simulink model "Aenea_model"  (R2020b)
settings: Solver=FixedStepDiscrete  StartTime=0.0  StopTime=10.0  FixedStep=0.02  RelTol=1e-3
undefined symbols (not defined in the file or in its folder): attuatore_Amax, attuatore_Amin, attuatore_Emax, attuatore_Emin, attuatore_Rmax, attuatore_Rmin, attuatore_Tmax, attuatore_Tmin, bias, DiscIntNeverNeededParam, interventoA_05, interventoA_1, interventoE_05, interventoE_1, interventoT, inv_A, inv_comp_h, inv_E, inv_R, inv_T, K_AW_B_AP_quota, K_AW_B_becc, K_AW_B_imb, K_AW_B_roll, K_imb_inv, Kd_h_app, Kd_h_flare, Ki_AP_quota_select, Ki_AP_rotta, Ki_AP_vel, Ki_becch, Ki_h_app, Ki_h_cruise, Ki_h_flare, Ki_roll, Kp_AP_quota_hold_h, Kp_AP_quota_hold_l, Kp_AP_quota_select, Kp_AP_rotta, Kp_AP_vel, Kp_becch, Kp_comp_h, Kp_h_app_max, Kp_h_app_min, Kp_h_cruise, Kp_h_flare, Kp_imb, Kp_p, Kp_q, Kp_roll, Kp_Rotta_ATO, Newton, phi_max, phi_min, Q1B, R1B, Raphson, safe_phi, safe_V, Sensor_Offsets ... (+11)
libraries: simulink_extras x41, slpidlib x8, simulink x6, dspsigops x4, arduinolib x3, svdutilitieslib x3, aerolibtransform2sys x2, aerolibtransform2 x2, aerosimlib x2, cstblocks x1
(part 4 of 7)

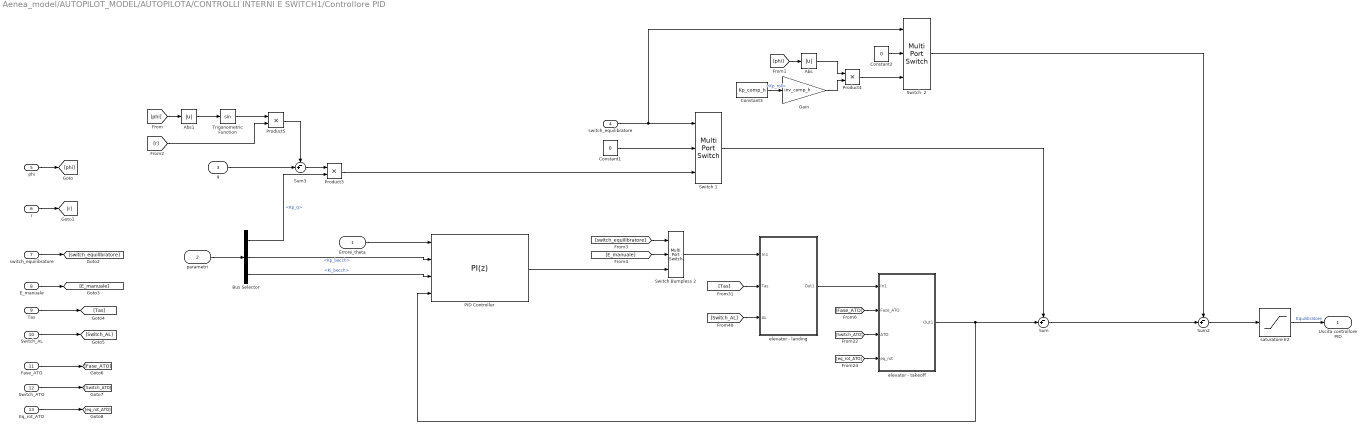
== system Aenea_model/AUTOPILOT_MODEL/AUTOPILOTA/CONTROLLI INTERNI E SWITCH1/Controllore PID ==
  Errore_theta : Inport
  parametri : Inport  Port=2
  "q " : Inport  Port=3
  "switch_equilibratore " : Inport  Port=4
  "phi " : Inport  Port=5
  r : Inport  Port=6
  switch_equilibratore : Inport  Port=7
  E_manuale : Inport  Port=8
  Tas : Inport  Port=9
  Switch_AL : Inport  Port=10
  Fase_ATO : Inport  Port=11
  Switch_ATO : Inport  Port=12
  Eq_rot_ATO : Inport  Port=13
  Abs : Abs
  Abs1 : Abs
  Bus Selector : BusSelector  OutputSignals=Kp_q,Kp_becch,Ki_becch
  Constant1 : Constant  Value=0  SampleTime=0.02
  Constant2 : Constant  Value=0  SampleTime=0.02
  Constant3 : Constant  Value=Kp_comp_h  SampleTime=0.02
  Gain : Gain  Gain=inv_comp_h
  PID Controller : slpidlib/PID Controller  Controller=PI  Form=Parallel  TimeDomain=Discrete-time  UseExternalTs=off  SampleTime=-1  IntegratorMethod=Forward Euler  FilterMethod=Forward Euler  ControllerParametersSource=external  P=1  I=1  D=1  UseFilter=off  N=100  TunerSelectOption=Transfer Function Based (PID Tuner App)  InitialConditionSource=internal  InitialConditionForIntegrator=0  InitialConditionForFilter=0  DifferentiatorICPrevScaledInput=0  ExternalReset=none  TrackingMode=on  Kt=1  LimitOutput=on  SatLimitsSource=internal  UpperSaturationLimit=attuatore_Emax  LowerSaturationLimit=attuatore_Emin  LinearizeAsGain=on  AntiWindupMode=back-calculation  Kb=1  POutMin=[]  POutMax=[]  IOutMin=[]  IOutMax=[]  DOutMin=[]  DOutMax=[]  NOutMin=[]  NOutMax=[]  SumOutMin=[]  SumOutMax=[]  SaturationOutMin=[]  SaturationOutMax=[]  PParamMin=[]  PParamMax=[]  IParamMin=[]  IParamMax=[]  DParamMin=[]  DParamMax=[]  NParamMin=[]  NParamMax=[]  KbParamMin=[]  KbParamMax=[]  KtParamMin=[]  KtParamMax=[]  KbOutMin=[]  KbOutMax=[]  KtOutMin=[]  KtOutMax=[]  IntegratorOutMin=[]  IntegratorOutMax=[]  FilterOutMin=[]  FilterOutMax=[]  SumI1OutMin=[]  SumI1OutMax=[]  SumI2OutMin=[]  SumI2OutMax=[]  SumI3OutMin=[]  SumI3OutMax=[]  SumI4OutMin=[]  SumI4OutMax=[]  SumDOutMin=[]  SumDOutMax=[]  DifferentiatorOutMin=[]  DifferentiatorOutMax=[]  FilterDiffOutCoefMin=[]  FilterDiffOutCoefMax=[]  ReciprocalOutMin=[]  ReciprocalOutMax=[]  SumDenOutMin=[]  SumDenOutMax=[]  SumNumOutMin=[]  SumNumOutMax=[]  DivideOutMin=[]  DivideOutMax=[]  UdiffTsProdOutMin=[]  UdiffTsProdOutMax=[]  NTsProdOutMin=[]  NTsProdOutMax=[]  UintegralTsProdOutMin=[]  UintegralTsProdOutMax=[]  UngainTsProdOutMin=[]  UngainTsProdOutMax=[]  IntegratorContinuousStateAttributes=''  IntegratorStateMustResolveToSignalObject=off  IntegratorRTWStateStorageClass=Auto  FilterContinuousStateAttributes=''  FilterStateMustResolveToSignalObject=off  FilterRTWStateStorageClass=Auto  ParallelPVariant=ExternalParameters  IdealPVariant=Disabled  IVariant=ExternalParameters  DVariant=Disabled  IntegratorVariant=Discrete  SatVariant=Enabled  AWVariant=BackCalculation  PCopyVariant=Disabled  TRVariant=Enabled  FdbkBlocksVariant=Forward  IdealPFdbkVariant=Disabled  SatFdbkVariant=Disabled  DerivativeFilterVariant=Disabled  NVariant=Disabled  NCopyVariant=Disabled_SignalSpec  FilterICVariant=Disabled  IntegratorICVariant=InternalICs  ExternalResetVariant=Disabled  TRSumVariant=TrackingMode  SumFdbkVariant=Disabled  SumVariant=Sum_PI  TsampFilterVariant=InternalTs  TsampNgainVariant=Passthrough  TsampIntegralVariant=Passthrough  ExternalSaturationOutDataTypeStr=Inherit: Same as second input
  Product3 : Product  RndMeth=Zero
  Product4 : Product  RndMeth=Zero
  Product5 : Product  RndMeth=Zero
  Sum : Sum  Inputs=-+|
  Sum2 : Sum  Inputs=-+|
  Sum3 : Sum  Inputs=-+|
  Switch  2 : MultiPortSwitch  DataPortOrder=Zero-based contiguous  Inputs=2  zeroidx=on
  Switch 1 : MultiPortSwitch  DataPortOrder=Zero-based contiguous  Inputs=2  zeroidx=on
  Switch Bumpless 2 : MultiPortSwitch  DataPortOrder=Zero-based contiguous  Inputs=2  zeroidx=on
  Trigonometric Function : Trigonometry
  elevator - landing : Subsystem
  elevator - takeoff : Subsystem
  saturatore E2 : Saturate  UpperLimit=attuatore_Emax  LowerLimit=attuatore_Emin
  Uscita controllore PID : Outport  VectorParamsAs1DForOutWhenUnconnected=off
  wires:
  Errore_theta/1 -> PID Controller/1
  parametri/1 -> Bus Selector/1
  Bus Selector/2 -> PID Controller/2  "<Kp_becch>"
  Bus Selector/3 -> PID Controller/3  "<Ki_becch>"
  Bus Selector/1 -> Product3/2  "<Kp_q>"
  Switch 1/1 -> Sum/1
  Product3/1 -> Switch 1/3
  Constant1/1 -> Switch 1/2
  elevator - takeoff/1(Out1) -> PID Controller/4, Sum/2
  Sum2/1 -> saturatore E2/1
  [phi] -> Abs/1
  Switch  2/1 -> Sum2/1
  Product4/1 -> Switch  2/3
  Constant2/1 -> Switch  2/2
  "switch_equilibratore "/1 -> Switch  2/1, Switch 1/1
  Abs/1 -> Product4/1
  [phi] -> Abs1/1
  Abs1/1 -> Trigonometric Function/1
  "phi "/1 -> [phi]
  r/1 -> [r]
  Trigonometric Function/1 -> Product5/1
  [r] -> Product5/2
  "q "/1 -> Sum3/2
  Sum3/1 -> Product3/1
  Product5/1 -> Sum3/1
  Sum/1 -> Sum2/2
  Switch Bumpless 2/1 -> elevator - landing/1(In1)
  Gain/1 -> Product4/2
  [Tas] -> elevator - landing/2(Tas)
  [Switch_AL] -> elevator - landing/3(AL)
  [Switch_ATO] -> elevator - takeoff/3(ATO)
  [Fase_ATO] -> elevator - takeoff/2(Fase_ATO)
  [eq_rot_ATO] -> elevator - takeoff/4(eq_rot)
  elevator - landing/1(Out1) -> elevator - takeoff/1(In1)
  [E_manuale] -> Switch Bumpless 2/2
  PID Controller/1 -> Switch Bumpless 2/3
  [switch_equilibratore] -> Switch Bumpless 2/1
  switch_equilibratore/1 -> [switch_equilibratore]
  E_manuale/1 -> [E_manuale]
  Tas/1 -> [Tas]
  Switch_AL/1 -> [Switch_AL]
  Fase_ATO/1 -> [Fase_ATO]
  Switch_ATO/1 -> [Switch_ATO]
  Eq_rot_ATO/1 -> [eq_rot_ATO]
  saturatore E2/1 -> Uscita controllore PID/1  "Equilibratore"
  Constant3/1 -> Gain/1  "<Kp_roll>"

== system Aenea_model/AUTOPILOT_MODEL/AUTOPILOTA/CONTROLLI INTERNI E SWITCH1/Controllore PID1 ==
  Err_Trk : Inport
  Errore_phi : Inport  Port=2
  parametri : Inport  Port=3
  "p " : Inport  Port=4
  "switch_alettoni " : Inport  Port=5
  Fase_ATO : Inport  Port=6
  Bus Selector : BusSelector  OutputSignals=Kp_p,Kp_roll,Ki_roll
  Constant1 : Constant  Value=0  SampleTime=0.02
  Constant3 : Constant  Value=2
  PID Controller : slpidlib/PID Controller  Controller=PI  Form=Parallel  TimeDomain=Discrete-time  UseExternalTs=off  SampleTime=0.02  IntegratorMethod=Forward Euler  FilterMethod=Forward Euler  ControllerParametersSource=external  P=1  I=1  D=0  UseFilter=on  N=100  TunerSelectOption=Transfer Function Based (PID Tuner App)  InitialConditionSource=internal  InitialConditionForIntegrator=0  InitialConditionForFilter=0  DifferentiatorICPrevScaledInput=0  ExternalReset=rising  TrackingMode=on  Kt=1  LimitOutput=on  SatLimitsSource=internal  UpperSaturationLimit=attuatore_Amax  LowerSaturationLimit=attuatore_Amin  LinearizeAsGain=on  AntiWindupMode=back-calculation  Kb=0.5  POutMin=[]  POutMax=[]  IOutMin=[]  IOutMax=[]  DOutMin=[]  DOutMax=[]  NOutMin=[]  NOutMax=[]  SumOutMin=[]  SumOutMax=[]  SaturationOutMin=[]  SaturationOutMax=[]  PParamMin=[]  PParamMax=[]  IParamMin=[]  IParamMax=[]  DParamMin=[]  DParamMax=[]  NParamMin=[]  NParamMax=[]  KbParamMin=[]  KbParamMax=[]  KtParamMin=[]  KtParamMax=[]  KbOutMin=[]  KbOutMax=[]  KtOutMin=[]  KtOutMax=[]  IntegratorOutMin=[]  IntegratorOutMax=[]  FilterOutMin=[]  FilterOutMax=[]  SumI1OutMin=[]  SumI1OutMax=[]  SumI2OutMin=[]  SumI2OutMax=[]  SumI3OutMin=[]  SumI3OutMax=[]  SumI4OutMin=[]  SumI4OutMax=[]  SumDOutMin=[]  SumDOutMax=[]  DifferentiatorOutMin=[]  DifferentiatorOutMax=[]  FilterDiffOutCoefMin=[]  FilterDiffOutCoefMax=[]  ReciprocalOutMin=[]  ReciprocalOutMax=[]  SumDenOutMin=[]  SumDenOutMax=[]  SumNumOutMin=[]  SumNumOutMax=[]  DivideOutMin=[]  DivideOutMax=[]  UdiffTsProdOutMin=[]  UdiffTsProdOutMax=[]  NTsProdOutMin=[]  NTsProdOutMax=[]  UintegralTsProdOutMin=[]  UintegralTsProdOutMax=[]  UngainTsProdOutMin=[]  UngainTsProdOutMax=[]  IntegratorContinuousStateAttributes=''  IntegratorStateMustResolveToSignalObject=off  IntegratorRTWStateStorageClass=Auto  FilterContinuousStateAttributes=''  FilterStateMustResolveToSignalObject=off  FilterRTWStateStorageClass=Auto  ParallelPVariant=ExternalParameters  IdealPVariant=Disabled  IVariant=ExternalParameters  DVariant=Disabled  IntegratorVariant=Discrete  SatVariant=Enabled  AWVariant=BackCalculation  PCopyVariant=Disabled  TRVariant=Enabled  FdbkBlocksVariant=Forward  IdealPFdbkVariant=Disabled  SatFdbkVariant=Disabled  DerivativeFilterVariant=Disabled  NVariant=Disabled  NCopyVariant=Disabled_SignalSpec  FilterICVariant=Disabled  IntegratorICVariant=InternalICs  ExternalResetVariant=ExternalReset  TRSumVariant=TrackingMode  SumFdbkVariant=Disabled  SumVariant=Sum_PI  TsampFilterVariant=InternalTs  TsampNgainVariant=Passthrough  TsampIntegralVariant=Passthrough  ExternalSaturationOutDataTypeStr=Inherit: Same as second input
  Product3 : Product  RndMeth=Zero
  Sum : Sum  Inputs=|+-
  Sum2 : Sum  Inputs=-+|
  Switch Bumpless 1 : MultiPortSwitch  DataPortOrder=Zero-based contiguous  Inputs=2  zeroidx=on
  Uscita controllore PID : Outport  VectorParamsAs1DForOutWhenUnconnected=off
  wires:
  Errore_phi/1 -> PID Controller/1
  parametri/1 -> Bus Selector/1
  Bus Selector/2 -> PID Controller/2  "<Kp_roll>"
  Bus Selector/3 -> PID Controller/3  "<Ki_roll>"
  "p "/1 -> Product3/1
  Switch Bumpless 1/1 -> Sum2/1
  Product3/1 -> Switch Bumpless 1/3
  "switch_alettoni "/1 -> Switch Bumpless 1/1
  Constant1/1 -> Switch Bumpless 1/2
  Bus Selector/1 -> Product3/2  "<Kp_p>"
  Sum2/1 -> Uscita controllore PID/1
  PID Controller/1 -> Sum2/2
  Err_Trk/1 -> PID Controller/5
  Fase_ATO/1 -> Sum/1
  Constant3/1 -> Sum/2
  Sum/1 -> PID Controller/4

== system Aenea_model/AUTOPILOT_MODEL/AUTOPILOTA/CONTROLLI INTERNI E SWITCH1/Filtro Washout1 ==
  In : Inport
  Discrete Washout Filter : DiscreteTransferFcn  Numerator=[ 1 -1]  Denominator=[1 -0.995]  SampleTime=t_AP
  Discrete Washout Filter1 : DiscreteTransferFcn  Commented=on  Numerator=[1.234 -1.234]  Denominator=[1 -0.995]  SampleTime=tsamp
  Out : Outport  VectorParamsAs1DForOutWhenUnconnected=off
  wires:
  In/1 -> Discrete Washout Filter/1
  Discrete Washout Filter/1 -> Out/1

== system Aenea_model/AUTOPILOT_MODEL/AUTOPILOTA/CONTROLLI INTERNI E SWITCH1/manetta - takeoff ==
  note: Quando verra caricato sull'autopilota bisogna modificare il limite del saturatore e metterlo ad 1
  In1 : Inport
  Fase_ATO : Inport  Port=2
  ATO : Inport  Port=3
  manetta_ref_ATO : Inport  Port=4
  Constant4 : Constant  Value=0
  Constant7 : Constant  Value=10
  Constant8 : Constant
  Discrete-Time Integrator : DiscreteIntegrator  gainval=0.015  ExternalReset=rising  SampleTime=-1  LimitOutput=on  UpperSaturationLimit=0.6  LowerSaturationLimit=0  ICPrevOutput=DiscIntNeverNeededParam  ICPrevScaledInput=DiscIntNeverNeededParam
  Multiport Switch1 : MultiPortSwitch  DataPortOrder=Zero-based contiguous  Inputs=2  zeroidx=on
  Sum : Sum  Inputs=|+-
  Switch Bumpless 1 : MultiPortSwitch  DataPortOrder=Zero-based contiguous  Inputs=5  zeroidx=on
  Out1 : Outport  VectorParamsAs1DForOutWhenUnconnected=off
  wires:
  Discrete-Time Integrator/1 -> Switch Bumpless 1/4
  Constant7/1 -> Discrete-Time Integrator/1
  Constant8/1 -> Sum/2
  manetta_ref_ATO/1 -> Switch Bumpless 1/3
  Constant4/1 -> Switch Bumpless 1/2
  ATO/1 -> Multiport Switch1/1
  Switch Bumpless 1/1 -> Multiport Switch1/3
  Sum/1 -> Discrete-Time Integrator/2
  In1/1 -> Multiport Switch1/2, Switch Bumpless 1/5, Switch Bumpless 1/6  "Manetta"
  Fase_ATO/1 -> Switch Bumpless 1/1, Sum/1
  Multiport Switch1/1 -> Out1/1  "Manetta"

== system Aenea_model/AUTOPILOT_MODEL/AUTOPILOTA/GESTIONE AUTOPILOTI1/Interruttore_Intervento ==
  note: Quando si preme il pulsante per il test dell'intervento pilota su QGC int_sw_intervento = 1 e si attiva l'Enabled Subsystem, quando si riva in manual int_sw_intervento torna a zero e il subsystem non si attiva. Inoltre contemporaneamente ogni volta che int_sw_intervento da 0 passa a 1 si attiva anche il Resettable Subsystem che resetta il clock che altrimenti continuerebbe a contare e non permetterebbe di rifare il test una seconda volta dato che L'Enable Subsystem restituirebbe 0.
  note: Quando è attivo manda un 1 per due secondi e poi 0.
  int_sw_intervento : Inport
  Display : Display
  Display1 : Display
  Enabled Subsystem : Subsystem  TreatAsAtomicUnit=on
  Resettable Subsystem : Subsystem  TreatAsAtomicUnit=on
  1/0 : Outport  VectorParamsAs1DForOutWhenUnconnected=off
  wires:
  int_sw_intervento/1 -> Resettable Subsystem/Reset, Enabled Subsystem/Enable, Display1/1
  Enabled Subsystem/1(1/0) -> Display/1, 1/0/1
  Resettable Subsystem/1(Time) -> Enabled Subsystem/1(Time)

== system Aenea_model/AUTOPILOT_MODEL/AUTOPILOTA/GESTIONE AUTOPILOTI1/Interruttore_Safe ==
  note: Quando si preme il pulsante per il test del SAFE su QGC int_sw_safe = 1 e si attiva l'Enabled Subsystem, quando si riva in manual int_sw_safe torna a zero e il subsystem non si attiva. Inoltre contemporaneamente ogni volta che int_sw_sefe da 0 passa
      | a 1 si attiva anche il Resettable Subsystem che resetta il clock che altrimenti continuerebbe a contare e non permetterebbe di rifare il test una seconda volta dato che L'Enable Subsystem restituirebbe 0.
  note: Quando è attivo manda un 1 per due secondi e poi 0.
  int_sw_safe : Inport
  Enabled Subsystem : Subsystem  TreatAsAtomicUnit=on
  Resettable Subsystem : Subsystem  TreatAsAtomicUnit=on
  1/0 : Outport  VectorParamsAs1DForOutWhenUnconnected=off
  wires:
  int_sw_safe/1 -> Resettable Subsystem/Reset, Enabled Subsystem/Enable
  Enabled Subsystem/1(1/0) -> 1/0/1
  Resettable Subsystem/1(Time) -> Enabled Subsystem/1(Time)

== system Aenea_model/AUTOPILOT_MODEL/AUTOPILOTA/GESTIONE AUTOPILOTI1/Intervento Manager ==
  Manuale : Inport
  Ingaggio_AP : Inport  Port=2
  absE : Inport  Port=3
  absA : Inport  Port=4
  absT : Inport  Port=5
  Alarm_Timing_0.5sec : Subsystem
  Alarm_Timing_1sec : Subsystem
  Constant : Constant  Value=interventoE_1
  Constant1 : Constant  Value=interventoE_05
  Constant2 : Constant  Value=interventoT
  Constant3 : Constant  Value=interventoA_1
  Constant4 : Constant  Value=interventoA_05
  MATLAB Function1 : MATLAB Function  TreatAsAtomicUnit=on
  Switch : Switch  Criteria=u2 ~= 0
  Alarm_Intervento : Outport  VectorParamsAs1DForOutWhenUnconnected=off
  wires:
  Switch/1 -> Alarm_Intervento/1
  Manuale/1 -> MATLAB Function1/1(Manuale)
  Ingaggio_AP/1 -> MATLAB Function1/2(Ingaggio_AP)
  absE/1 -> MATLAB Function1/3(absE)
  absA/1 -> MATLAB Function1/4(absA)
  absT/1 -> MATLAB Function1/5(absT)
  MATLAB Function1/2(sw) -> Switch/2
  MATLAB Function1/1(Int_1) -> Alarm_Timing_1sec/1(Intervento_IN)
  MATLAB Function1/3(Int_05) -> Alarm_Timing_0.5sec/1(Intervento_IN)
  Alarm_Timing_1sec/1(Alarm) -> Switch/1
  Alarm_Timing_0.5sec/1(Alarm) -> Switch/3
  Constant/1 -> MATLAB Function1/6(interventoE_1)
  Constant1/1 -> MATLAB Function1/7(interventoE_05)
  Constant2/1 -> MATLAB Function1/10(interventoT)
  Constant3/1 -> MATLAB Function1/8(interventoA_1)
  Constant4/1 -> MATLAB Function1/9(interventoA_05)

== system Aenea_model/AUTOPILOT_MODEL/AUTOPILOTA/GESTIONE AUTOPILOTI1/Safe Manager ==
  note: Quando si preme il tasto Test SAFE MODE su QGC la Matlab Function riceve un valore di Veloc = 50 per due sec
      | e quindi per due sec essa restituisce Alarm_safe = 1. Dato che tale valore persiste per due secondi il Subsystem
      | successivo pone Alarm_Safe = 1. Esso successivamente è inviato allo state flow.
  Veloc : Inport
  phi : Inport  Port=2
  ingaggio_AP : Inport  Port=3
  Manuale : Inport  Port=4
  Alarm_Timing : Subsystem
  Constant : Constant  Value=safe_V
  Constant1 : Constant  Value=safe_phi
  MATLAB Function1 : MATLAB Function  TreatAsAtomicUnit=on
  Alarm_Safe : Outport  VectorParamsAs1DForOutWhenUnconnected=off
  wires:
  Alarm_Timing/1(Alarm) -> Alarm_Safe/1
  Veloc/1 -> MATLAB Function1/1(Veloc)
  ingaggio_AP/1 -> MATLAB Function1/3(ingaggio_AP)
  phi/1 -> MATLAB Function1/2(phi)
  MATLAB Function1/1(Alarm_safe) -> Alarm_Timing/1(Alarm_IN)
  Constant/1 -> MATLAB Function1/4(safe_V)
  Constant1/1 -> MATLAB Function1/5(safe_phi)
  Manuale/1 -> MATLAB Function1/6(Manuale)

== system Aenea_model/AUTOPILOT_MODEL/AUTOPILOTA/GESTIONE AUTOPILOTI1/abs comandi manuali ==
  comandi manuali : Inport
  Abs{,1..3} (4 alike) : Abs
  Bus Creator : BusCreator  Inputs=4
  Bus Selector : BusSelector  OutputSignals=Manual Elevator,Manual Aileron,Manual Rudder,Manual Throttle
  Out : Outport  VectorParamsAs1DForOutWhenUnconnected=off
  wires:
  comandi manuali/1 -> Bus Selector/1
  Bus Selector/1 -> Abs/1  "<Manual Elevator>"
  Abs/1 -> Bus Creator/1  "abs_Manual Elevator"
  Bus Selector/2 -> Abs1/1  "<Manual Aileron>"
  Bus Selector/3 -> Abs2/1  "<Manual Rudder>"
  Bus Selector/4 -> Abs3/1  "<Manual Throttle>"
  Abs1/1 -> Bus Creator/2  "abs_Manual Aileron"
  Abs2/1 -> Bus Creator/3  "abs_Manual Rudder"
  Abs3/1 -> Bus Creator/4  "abs_Manual Throttle"
  Bus Creator/1 -> Out/1

== system Aenea_model/AUTOPILOT_MODEL/AUTOPILOTA/Subsystem1/DECOLLO AUTOMATICO ==
  Tas : Inport
  h : Inport  Port=2
  modo : Inport  Port=3
  psi_imu : Inport  Port=4
  theta : Inport  Port=5
  V_ : Inport  Port=6
  Enable : EnablePort
  Chart1 : Stateflow chart  TreatAsAtomicUnit=on
  Memory : Memory
  Memory1 : Memory
  Radians to Degrees : simulink_extras/Transformations/Radians to Degrees
  Radians to Degrees1 : simulink_extras/Transformations/Radians to Degrees
  Sample and Hold : dspsigops/Sample and Hold  trig=Rising edge  initCond=0  latchinput=off
  Sample and Hold1 : dspsigops/Sample and Hold  trig=Rising edge  initCond=0  latchinput=off
  rotta_ATO : Outport  VectorParamsAs1DForOutWhenUnconnected=off
  Fase_ATO : Outport  Port=2  VectorParamsAs1DForOutWhenUnconnected=off
  manetta_ref_ATO : Outport  Port=3  VectorParamsAs1DForOutWhenUnconnected=off
  eq_rot_ATO : Outport  Port=4  VectorParamsAs1DForOutWhenUnconnected=off
  phi_ref_ATO : Outport  Port=5  VectorParamsAs1DForOutWhenUnconnected=off
  theta_ref_ATO : Outport  Port=6  VectorParamsAs1DForOutWhenUnconnected=off
  h_ref_ATO : Outport  Port=7  VectorParamsAs1DForOutWhenUnconnected=off
  Tas_ref_ATO : Outport  Port=8  VectorParamsAs1DForOutWhenUnconnected=off
  RC_ref_ATO : Outport  Port=9  VectorParamsAs1DForOutWhenUnconnected=off
  wires:
  Chart1/3(psi_ref) -> rotta_ATO/1  "ROTTA"
  modo/1 -> Chart1/1(modo)
  h/1 -> Chart1/3(h)
  Tas/1 -> Chart1/2(TAS)
  Chart1/10(psi_ref_selector) -> Memory/1
  Memory/1 -> Sample and Hold/Trigger
  Sample and Hold/1 -> Chart1/4(psi_hold)
  psi_imu/1 -> Radians to Degrees1/1
  Chart1/1(Fase_ATO) -> Fase_ATO/1
  Chart1/2(manetta_ref) -> manetta_ref_ATO/1
  Chart1/7(h_ref) -> h_ref_ATO/1
  Chart1/4(eq_rot) -> eq_rot_ATO/1
  Chart1/5(phi_ref) -> phi_ref_ATO/1
  Chart1/6(pitch_ref) -> theta_ref_ATO/1
  Chart1/8(Tas_ref) -> Tas_ref_ATO/1
  Chart1/9(RC_ref) -> RC_ref_ATO/1
  Sample and Hold1/1 -> Chart1/5(theta_ground_hold)
  Chart1/11(theta_ground_selector) -> Memory1/1
  Memory1/1 -> Sample and Hold1/Trigger
  theta/1 -> Radians to Degrees/1
  Radians to Degrees/1 -> Sample and Hold1/1
  V_/1 -> Chart1/6(V_)
  Radians to Degrees1/1 -> Sample and Hold/1

== system Aenea_model/AUTOPILOT_MODEL/AUTOPILOTA/Subsystem1/Subsystem ==
  In1 : Inport
  In2 : Inport  Port=2
  In3 : Inport  Port=3
  In4 : Inport  Port=4
  In5 : Inport  Port=5
  <IAS> : Inport  Port=6
  In7 : Inport  Port=7
  <ALT> : Inport  Port=8
  <HDG> : Inport  Port=9
  In10 : Inport  Port=10
  <RC> : Inport  Port=11
  In12 : Inport  Port=12
  <Ingaggio_AP> : Inport  Port=13
  In14 : Inport  Port=14
  Enable : EnablePort
  Abs : Abs
  Data Type Conversion{,1..3} (4 alike) : DataTypeConversion  OutDataTypeStr=double
  Memory{,1..3,6} (5 alike) : Memory  InheritSampleTime=on
  Radians to Degrees3 : simulink_extras/Transformations/Radians to Degrees
  VETTORIALE : MATLAB Function  TreatAsAtomicUnit=on
  Out1 : Outport  VectorParamsAs1DForOutWhenUnconnected=off
  Out2 : Outport  Port=2  VectorParamsAs1DForOutWhenUnconnected=off
  Out3 : Outport  Port=3  VectorParamsAs1DForOutWhenUnconnected=off
  Out4 : Outport  Port=4  VectorParamsAs1DForOutWhenUnconnected=off
  wires:
  Data Type Conversion1/1 -> VETTORIALE/8(VELOCITA)
  Memory1/1 -> VETTORIALE/18(ALT_pre)
  VETTORIALE/5(ingaggio_AP_mem) -> Memory6/1
  Data Type Conversion2/1 -> VETTORIALE/9(QUOTA)
  VETTORIALE/8(ALT_pre_mem) -> Memory1/1
  Radians to Degrees3/1 -> VETTORIALE/11(HEADING)
  Memory6/1 -> VETTORIALE/15(ingaggio_AP_pre)
  In12/1 -> VETTORIALE/13(h)
  Memory3/1 -> VETTORIALE/16(modo_pre)
  VETTORIALE/6(modo_pre_mem) -> Memory3/1
  Abs/1 -> VETTORIALE/10(RC)
  VETTORIALE/9(HDG_pre_mem) -> Memory/1
  Data Type Conversion3/1 -> Abs/1
  Memory/1 -> VETTORIALE/19(HDG_pre)
  Data Type Conversion/1 -> VETTORIALE/7(ROTTA)
  Memory2/1 -> VETTORIALE/17(IAS_pre)
  VETTORIALE/7(IAS_pre_mem) -> Memory2/1
  VETTORIALE/3(rotta_vett) -> Out3/1
  In1/1 -> VETTORIALE/1(modo)
  <ALT>/1 -> VETTORIALE/3(ALT)
  <RC>/1 -> VETTORIALE/5(I_RC)
  In5/1 -> Data Type Conversion3/1
  In4/1 -> Data Type Conversion2/1
  <Ingaggio_AP>/1 -> VETTORIALE/6(ingaggio_AP)
  In10/1 -> VETTORIALE/12(TAS)
  In7/1 -> Radians to Degrees3/1
  In3/1 -> Data Type Conversion1/1
  VETTORIALE/1(V_vett) -> Out1/1
  VETTORIALE/2(h_vett) -> Out2/1
  <IAS>/1 -> VETTORIALE/2(IAS)
  In2/1 -> Data Type Conversion/1
  In14/1 -> VETTORIALE/14(RC_default)
  VETTORIALE/4(RC_vett) -> Out4/1
  <HDG>/1 -> VETTORIALE/4(HDG)

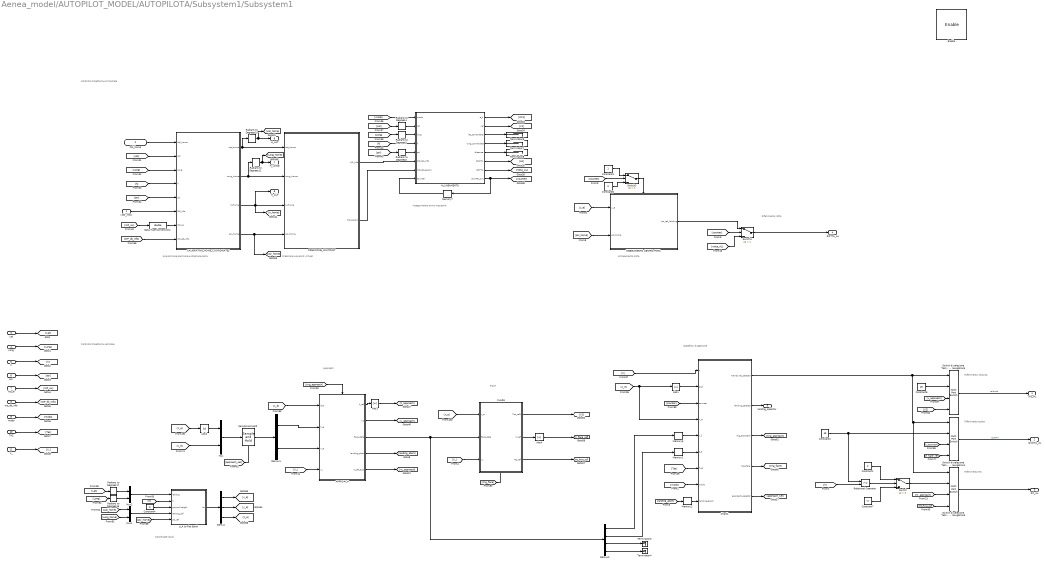
== system Aenea_model/AUTOPILOT_MODEL/AUTOPILOTA/Subsystem1/Subsystem1 ==
  note: Approach
  note: Controllo traiettoria verticale
  note: Flare
  note: Coordinate locali
  note: Stateflow di gestione
  note: Controllo traiettoria orizzontale
  note: Acquisizione posizione
      | e direzione pista
  note: Creazione waypoint
      | virtuali
  note: Inseguimento primo
      | waypoint
  note: Allineamento
      | pista
  note: Riferimento rotta
  note: Riferimento velocità
  note: Riferimento quota
  note: Riferimento RC
  <GC_info> : Inport
  Cal_home : Inport  Port=2
  Lat : Inport  Port=3
  Long : Inport  Port=4
  h : Inport  Port=5
  psi : Inport  Port=6
  wp_al : Inport  Port=7
  wp_db_info : Inport  Port=8
  modo : Inport  Port=9
  TAS : Inport  Port=10
  V_ : Inport  Port=11
  Enable : EnablePort
  ALLINEAMENTO : MATLAB Function  TreatAsAtomicUnit=on
  APPROACH : Subsystem
  Abs{1..4} (4 alike) : Abs
  CALIBRATING_HOME_COORDINATES : MATLAB Function  TreatAsAtomicUnit=on
  "CREAZIONE_WAYPOINT " : Subsystem
  Chart1 : Stateflow chart  TreatAsAtomicUnit=on
  Constant1 : Constant  Value=2  SampleTime=0.02
  Constant2 : Constant  Value=45  SampleTime=0.02
  Constant3 : Constant
  Constant4 : Constant  Value=0  SampleTime=0.02
  Constant6 : Constant  Value=20  SampleTime=0.02
  Constant7 : Constant  Value=-2  SampleTime=0.02
  Constant8 : Constant  Value=0
  Data Type Conversion4 : DataTypeConversion  OutDataTypeStr=double
  Demux : Demux  Outputs=3
  Demux1 : Demux  Outputs=2
  Demux2 : Demux
  FLARE : Subsystem
  INSEGUIMENTO CENTRO PISTA : Subsystem
  LLA to Flat Earth : Subsystem
  Memory1 : Memory
  Memory2 : Memory
  Memory5 : Memory
  Memory7 : Memory  InitialCondition=1  InheritSampleTime=on
  Mux : Mux  Inputs=2
  Mux1 : Mux  Inputs=2
  Mux2 : Mux  Inputs=2
  Radians to Degrees{4..6,10..11,16..17} (7 alike) : simulink_extras/Transformations/Radians to Degrees
  Relational Operator : RelationalOperator  OutDataTypeStr=boolean  RndMeth=Simplest
  Sample and Hold : dspsigops/Sample and Hold  trig=Rising edge  initCond=[0 0]  latchinput=off
  Switch : Switch  Criteria=u2 > Threshold
  Switch di selezione Task - Waypoint navigation4 : MultiPortSwitch
  Switch di selezione Task - Waypoint navigation5 : MultiPortSwitch
  Switch di selezione Task - Waypoint navigation6 : MultiPortSwitch
  Switch1 : Switch  Criteria=u2 > Threshold  Threshold=1
  Switch2 : Switch  Criteria=u2 > Threshold  Threshold=1
  Terminator{3..4,6..8} (5 alike) : Terminator
  TAS_AL : Outport  VectorParamsAs1DForOutWhenUnconnected=off
  QUOTA_AL : Outport  Port=2  VectorParamsAs1DForOutWhenUnconnected=off
  RC_AL : Outport  Port=3  VectorParamsAs1DForOutWhenUnconnected=off
  ROTTA_AL : Outport  Port=4  VectorParamsAs1DForOutWhenUnconnected=off
  landing_selector : Outport  Port=5  VectorParamsAs1DForOutWhenUnconnected=off
  H_LAT : Outport  Port=6  VectorParamsAs1DForOutWhenUnconnected=off
  H_LONG : Outport  Port=7  VectorParamsAs1DForOutWhenUnconnected=off
  H_ALT : Outport  Port=8  VectorParamsAs1DForOutWhenUnconnected=off
  wires:
  Chart1/1(maneuver_selector) -> Switch di selezione Task - Waypoint navigation6/1, Switch di selezione Task - Waypoint navigation4/1, Switch di selezione Task - Waypoint navigation5/1
  LLA to Flat Earth/1(Xe) -> Demux/1
  Radians to Degrees11/1 -> H_LONG/1, [Long_home]
  Mux/1 -> Sample and Hold/1
  ALLINEAMENTO/4(long_comandato) -> Terminator7/1
  Mux1/1 -> LLA to Flat Earth/4(latlong_ref)
  [WP_db_info] -> CALIBRATING_HOME_COORDINATES/8(WP_db_info)
  Demux1/2 -> APPROACH/3(x_g)
  Abs2/1 -> Mux/1
  ALLINEAMENTO/3(lat_comandato) -> Terminator6/1
  [rc_approach] -> Switch di selezione Task - Waypoint navigation6/3
  [V2] -> Switch di selezione Task - Waypoint navigation5/4
  [x_e] -> Chart1/4(x_e), Abs1/1
  Abs4/1 -> [h_flare_ref]
  CALIBRATING_HOME_COORDINATES/3(h_Home) -> H_ALT/1, [h_home], "CREAZIONE_WAYPOINT "/3(h_Home)
  [h] -> Chart1/1(h)
  [x_e] -> FLARE/1(x_e)
  [Long_home] -> Mux1/2
  APPROACH/3(flare_data) -> Demux2/1, FLARE/2(flare_data)
  CALIBRATING_HOME_COORDINATES/1(Lat_Home) -> Radians to Degrees10/1, "CREAZIONE_WAYPOINT "/1(Lat_Home)
  Demux/2 -> [y_e]
  FLARE/3(RC_ref) -> [RC_flare_ref]
  Chart1/4(trig_flare) -> [trig_flare]
  [h] -> LLA to Flat Earth/2(h)
  [Long] -> Radians to Degrees16/1
  Demux/3 -> [z_e]
  Demux2/2 -> Memory1/1
  Radians to Degrees10/1 -> H_LAT/1, [Lat_home]
  Sample and Hold/1 -> Demux1/1
  [trig_approach] -> APPROACH/Enable
  Switch/1 -> Switch di selezione Task - Waypoint navigation6/2
  Memory5/1 -> Chart1/5(x_f)
  Cal_home/1 -> CALIBRATING_HOME_COORDINATES/1(Cal_home)
  Demux2/3 -> Terminator3/1
  FLARE/2(h_ref) -> Abs4/1
  [z_e] -> Abs2/1
  [x_e] -> Mux/2
  CALIBRATING_HOME_COORDINATES/2(Long_Home) -> "CREAZIONE_WAYPOINT "/2(Long_Home), Radians to Degrees11/1
  Demux2/4 -> Terminator4/1
  FLARE/1(Tas_ref1) -> [V2]
  ALLINEAMENTO/7(ROTTA) -> [rotta_AL]
  APPROACH/2(V1) -> [v_approach]
  [V_] -> FLARE/3(V_)
  Chart1/5(approach_selector) -> [approach_sel]
  Abs1/1 -> Chart1/2(dist)
  [h_approach] -> Switch di selezione Task - Waypoint navigation4/3
  [RC_flare_ref] -> Switch di selezione Task - Waypoint navigation6/4
  Chart1/3(trig_approach) -> [trig_approach]
  [Lat_home] -> Mux1/1
  ALLINEAMENTO/6(QUOTA) -> [H1]
  ALLINEAMENTO/8(counter_out) -> Memory7/1, [counter]
  Demux/1 -> [x_e]
  Demux2/1 -> Memory5/1
  CALIBRATING_HOME_COORDINATES/4(psi_Home) -> [psi_home], "CREAZIONE_WAYPOINT "/4(psi_Home)
  Abs3/1 -> [h_approach]
  Mux2/1 -> LLA to Flat Earth/1(latlong)
  Chart1/2(landing_selector) -> landing_selector/1
  Constant2/1 -> Switch di selezione Task - Waypoint navigation4/2, Relational Operator/1
  [h_flare_ref] -> Switch di selezione Task - Waypoint navigation4/4
  [v_approach] -> Switch di selezione Task - Waypoint navigation5/3
  [Tas] -> Chart1/7(TAS)
  APPROACH/1(h_ref) -> Abs3/1
  Data Type Conversion4/1 -> CALIBRATING_HOME_COORDINATES/7(WP_AL)
  [Lat] -> Radians to Degrees17/1
  Demux1/1 -> APPROACH/2(h_g)
  Constant4/1 -> LLA to Flat Earth/3(ground height)
  [psi] -> CALIBRATING_HOME_COORDINATES/5(psi)
  ALLINEAMENTO/2(vel) -> [V1]
  Radians to Degrees5/1 -> ALLINEAMENTO/3(long)
  [x_e] -> APPROACH/1(dist)
  Memory7/1 -> ALLINEAMENTO/8(counter)
  [h] -> CALIBRATING_HOME_COORDINATES/4(h)
  [counter] -> Chart1/3(counter)
  Radians to Degrees4/1 -> ALLINEAMENTO/2(lat)
  [approach_sel] -> Sample and Hold/Trigger
  [Lat] -> Radians to Degrees4/1
  "CREAZIONE_WAYPOINT "/2(WP_param) -> ALLINEAMENTO/7(WP_db_param)
  [h] -> ALLINEAMENTO/4(h)
  [Long] -> Radians to Degrees5/1
  <GC_info>/1 -> CALIBRATING_HOME_COORDINATES/6(GC_info)
  ALLINEAMENTO/1(e_h) -> [RC1]
  Radians to Degrees6/1 -> ALLINEAMENTO/5(psi)
  Radians to Degrees16/1 -> Mux2/2
  [psi] -> Radians to Degrees6/1
  [WP_AL] -> Data Type Conversion4/1
  [modo] -> ALLINEAMENTO/1(modo)
  ALLINEAMENTO/5(distance) -> Terminator8/1
  Radians to Degrees17/1 -> Mux2/1
  "CREAZIONE_WAYPOINT "/1(WP_info) -> ALLINEAMENTO/6(WP_db_info)
  [trig_flare] -> FLARE/Enable
  Constant6/1 -> Switch di selezione Task - Waypoint navigation5/2
  [psi_home] -> LLA to Flat Earth/5(psi_ref)
  Switch di selezione Task - Waypoint navigation4/1 -> QUOTA_AL/1  "QUOTA"
  Switch di selezione Task - Waypoint navigation6/1 -> RC_AL/1
  Switch di selezione Task - Waypoint navigation5/1 -> TAS_AL/1  "velocita"
  Lat/1 -> [Lat]
  Long/1 -> [Long]
  h/1 -> [h]
  psi/1 -> [psi]
  wp_al/1 -> [WP_AL]
  wp_db_info/1 -> [WP_db_info]
  modo/1 -> [modo]
  TAS/1 -> [Tas]
  V_/1 -> [V_]
  Switch1/1 -> ROTTA_AL/1
  [h] -> Relational Operator/2
  Relational Operator/1 -> Switch/2
  Constant1/1 -> Switch/1
  Constant7/1 -> Switch/3
  [modo] -> Chart1/8(modo)
  APPROACH/4(landing_abort) -> [landing_abort]
  Memory1/1 -> Chart1/6(h_f)
  Memory2/1 -> Chart1/9(landing_abort)
  [landing_abort] -> Memory2/1
  [Lat] -> CALIBRATING_HOME_COORDINATES/2(Lat)
  [Long] -> CALIBRATING_HOME_COORDINATES/3(Long)
  [counter] -> Switch2/2
  [rotta_AL] -> Switch1/3
  [psi_home] -> INSEGUIMENTO CENTRO PISTA/2(psi_home)
  INSEGUIMENTO CENTRO PISTA/1(psi_ref_landing) -> Switch1/1
  [y_e] -> INSEGUIMENTO CENTRO PISTA/1(y_e)
  [counter] -> Switch1/2
  Constant8/1 -> Switch2/3
  Switch2/1 -> INSEGUIMENTO CENTRO PISTA/Enable
  Constant3/1 -> Switch2/1
  [V_] -> APPROACH/4(V_)
  APPROACH/5(rc_ref_app) -> [rc_approach]

== system Aenea_model/AUTOPILOT_MODEL/AUTOPILOTA/Subsystem1/Subsystem2 ==
  In1 : Inport
  In2 : Inport  Port=2
  In3 : Inport  Port=3
  In4 : Inport  Port=4
  In5 : Inport  Port=5
  In6 : Inport  Port=6
  <GC_info> : Inport  Port=7
  Enable : EnablePort
  Memory4 : Memory  InitialCondition=1  InheritSampleTime=on
  Radians to Degrees : simulink_extras/Transformations/Radians to Degrees
  Radians to Degrees1 : simulink_extras/Transformations/Radians to Degrees
  Radians to Degrees2 : simulink_extras/Transformations/Radians to Degrees
  Terminator : Terminator
  Terminator1 : Terminator
  Terminator2 : Terminator
  WAYPOINTS : MATLAB Function  TreatAsAtomicUnit=on
  saturatore V : Saturate  UpperLimit=40  LowerLimit=15
  saturatore V1 : Saturate  UpperLimit=2  LowerLimit=-2
  RC : Outport  VectorParamsAs1DForOutWhenUnconnected=off
  VELOCITA : Outport  Port=2  VectorParamsAs1DForOutWhenUnconnected=off
  Out3 : Outport  Port=3  VectorParamsAs1DForOutWhenUnconnected=off
  Out4 : Outport  Port=4  VectorParamsAs1DForOutWhenUnconnected=off
  wires:
  WAYPOINTS/8(counter_out) -> Memory4/1
  saturatore V1/1 -> RC/1  "RC"
  Radians to Degrees1/1 -> WAYPOINTS/2(long)
  WAYPOINTS/4(long_comandato) -> Terminator1/1
  Radians to Degrees/1 -> WAYPOINTS/1(lat)
  WAYPOINTS/2(vel) -> saturatore V/1
  WAYPOINTS/1(e_h) -> saturatore V1/1
  WAYPOINTS/5(distance) -> Terminator2/1
  WAYPOINTS/3(lat_comandato) -> Terminator/1
  Radians to Degrees2/1 -> WAYPOINTS/4(psi)
  Memory4/1 -> WAYPOINTS/8(counter)
  In1/1 -> Radians to Degrees/1
  In3/1 -> WAYPOINTS/3(h)
  In4/1 -> Radians to Degrees2/1
  In2/1 -> Radians to Degrees1/1
  WAYPOINTS/7(ROTTA) -> Out4/1
  In5/1 -> WAYPOINTS/5(WP_db_info)
  In6/1 -> WAYPOINTS/6(WP_db_param)
  <GC_info>/1 -> WAYPOINTS/7(GC_info)
  saturatore V/1 -> VELOCITA/1  "VELOCITA"
  WAYPOINTS/6(QUOTA) -> Out3/1

== system Aenea_model/AUTOPILOT_MODEL/AUTOPILOTA/Subsystem1/Subsystem3 ==
  In1 : Inport
  In2 : Inport  Port=2
  In3 : Inport  Port=3
  In4 : Inport  Port=4
  In5 : Inport  Port=5
  In6 : Inport  Port=6
  In7 : Inport  Port=7
  In8 : Inport  Port=8
  Enable : EnablePort
  GO_HOME : MATLAB Function  TreatAsAtomicUnit=on
  Radians to Degrees12 : simulink_extras/Transformations/Radians to Degrees
  Radians to Degrees13 : simulink_extras/Transformations/Radians to Degrees
  Radians to Degrees9 : simulink_extras/Transformations/Radians to Degrees
  Out1 : Outport  VectorParamsAs1DForOutWhenUnconnected=off
  Out2 : Outport  Port=2  VectorParamsAs1DForOutWhenUnconnected=off
  Out3 : Outport  Port=3  VectorParamsAs1DForOutWhenUnconnected=off
  Out4 : Outport  Port=4  VectorParamsAs1DForOutWhenUnconnected=off
  wires:
  GO_HOME/1(V_goHome) -> Out1/1
  GO_HOME/4(rotta_goHome) -> Out4/1
  GO_HOME/3(RC_goHome) -> Out3/1
  Radians to Degrees9/1 -> GO_HOME/4(psi)
  Radians to Degrees12/1 -> GO_HOME/1(lat)
  In2/1 -> Radians to Degrees13/1
  Radians to Degrees13/1 -> GO_HOME/2(long)
  In3/1 -> GO_HOME/3(h)
  In4/1 -> Radians to Degrees9/1
  In6/1 -> GO_HOME/6(Long_Home)
  In8/1 -> GO_HOME/8(V_goHome_rif)
  In5/1 -> GO_HOME/5(Lat_Home)
  In1/1 -> Radians to Degrees12/1
  GO_HOME/2(h_goHome) -> Out2/1
  In7/1 -> GO_HOME/7(h_goHome_rif)

== system Aenea_model/AUTOPILOT_MODEL/MISURE DA SENSORI FILTRATE/TRA 0-360/Subsystem1 ==
  +-180 : Inport
  Constant : Constant  Value=360
  Gain : Gain  Gain=-1
  Sum : Sum  Inputs=|++
  Switch : Switch  Criteria=u2 > Threshold
  0-360 : Outport  VectorParamsAs1DForOutWhenUnconnected=off
  wires:
  Constant/1 -> Sum/2
  +-180/1 -> Gain/1, Switch/3, Sum/1
  Gain/1 -> Switch/2
  Sum/1 -> Switch/1
  Switch/1 -> 0-360/1

== system Aenea_model/AUTOPILOT_MODEL/MISURE DA SENSORI FILTRATE/initializer//Clk_generator 2/Clock GPS1 ==
  In2 : Inport
  AND : Logic  Commented=on  IconShape=distinctive  AllPortsSameDT=off  OutDataTypeStr=boolean
  Equal1 : RelationalOperator  Operator===  OutDataTypeStr=boolean  RndMeth=Simplest
  From9 : From  Commented=on  GotoTag=mario
  MATLAB Function : MATLAB Function  TreatAsAtomicUnit=on
  MATLAB Function1 : MATLAB Function  TreatAsAtomicUnit=on
  Memory : Memory
  NOT : Logic  Operator=NOT  IconShape=distinctive  AllPortsSameDT=off  OutDataTypeStr=boolean
  NOT1 : Logic  Commented=on  Operator=NOT  IconShape=distinctive  AllPortsSameDT=off  OutDataTypeStr=boolean
  Pulse Generator3 : DiscretePulseGenerator  Commented=on  PulseType=Time based  Period=0.2  PulseWidth=10
  Terminator : Terminator  Commented=on
  clk_pos : Outport  VectorParamsAs1DForOutWhenUnconnected=off
  clk_vel : Outport  Port=2  VectorParamsAs1DForOutWhenUnconnected=off
  wires:
  Equal1/1 -> NOT/1
  NOT/1 -> MATLAB Function1/1(u), MATLAB Function/1(u)
  In2/1 -> Equal1/1, Memory/1
  Memory/1 -> Equal1/2
  From9/1 -> NOT1/1
  Pulse Generator3/1 -> AND/1
  NOT1/1 -> AND/2
  AND/1 -> Terminator/1
  MATLAB Function1/1(y) -> clk_pos/1
  MATLAB Function/1(y) -> clk_vel/1

== system Aenea_model/AUTOPILOT_MODEL/MISURE DA SENSORI FILTRATE/initializer//Clk_generator 2/Clock Mti ==
  In2 : Inport
  Equal : RelationalOperator  Operator===  OutDataTypeStr=boolean  RndMeth=Simplest
  MATLAB Function : MATLAB Function  TreatAsAtomicUnit=on
  Memory : Memory
  NOT : Logic  Operator=NOT  IconShape=distinctive  AllPortsSameDT=off  OutDataTypeStr=boolean
  Out1 : Outport  VectorParamsAs1DForOutWhenUnconnected=off
  wires:
  In2/1 -> Memory/1, Equal/1
  Equal/1 -> NOT/1
  Memory/1 -> Equal/2
  MATLAB Function/1(y) -> Out1/1
  NOT/1 -> MATLAB Function/1(u)

== system Aenea_model/AUTOPILOT_MODEL/Misure Sensori/ATTOPILOT/Scalatura_bit_to_percent_Volt ==
  Bit : Inport
  Sum : Sum  Inputs=|++
  m_attopilota_bit_to_percent : Gain  Gain=100/361  ParamDataTypeStr=double
  q_attopilota_bit_to_percent : Constant  Value=-204800/361
  Percent_Volt : Outport  VectorParamsAs1DForOutWhenUnconnected=off
  wires:
  Bit/1 -> m_attopilota_bit_to_percent/1
  Sum/1 -> Percent_Volt/1
  q_attopilota_bit_to_percent/1 -> Sum/2
  m_attopilota_bit_to_percent/1 -> Sum/1

== system Aenea_model/AUTOPILOT_MODEL/Misure Sensori/BMP_280/Dynamic rate limiter ==
  note: Y(k)
  note: U(k)
  up : Inport
  u : Inport  Port=2
  lo : Inport  Port=3
  Delay Input2 : UnitDelay  Description=Store in Global RAM  DisableCoverage=on  InitialCondition=101325  SampleTime=-1  HasFrameUpgradeWarning=on
  Difference Inputs1 : Sum  Description=Add in CPU  DisableCoverage=on  Inputs=+-  OutDataTypeStr=Inherit: Inherit via back propagation
  Difference Inputs2 : Sum  Description=Add in CPU  OutDataTypeStr=Inherit: Inherit via back propagation
  FixPt Data Type Duplicate : DataTypeDuplicate  DisableCoverage=on  NumInputPorts=7
  Saturation Dynamic : simulink/Discontinuities/Saturation Dynamic  OutMin=[]  OutMax=[]  OutDataTypeStr=Inherit: Same as second input  OutDataType=fixdt(1, 16)  OutScaling=2^-10  DoSatur=off
  delta fall limit : Product  DisableCoverage=on  Inputs=**  OutDataTypeStr=Inherit: Inherit via back propagation  SaturateOnIntegerOverflow=on
  delta rise limit : Product  DisableCoverage=on  Inputs=**  OutDataTypeStr=Inherit: Inherit via back propagation  SaturateOnIntegerOverflow=on
  sample time : SampleTimeMath  DisableCoverage=on  TsampMathOp=Ts Only  weightValue=1
  Y : Outport  InitialOutput=0  VectorParamsAs1DForOutWhenUnconnected=off
  wires:
  delta fall limit/1 -> Saturation Dynamic/3, FixPt Data Type Duplicate/3
  sample time/1 -> delta rise limit/2, delta fall limit/2
  lo/1 -> delta fall limit/1
  u/1 -> sample time/1, FixPt Data Type Duplicate/5, Difference Inputs1/1
  Difference Inputs1/1 -> Saturation Dynamic/2, FixPt Data Type Duplicate/4  "( U(k) - Y(k-1) )"
  Delay Input2/1 -> Difference Inputs2/2, FixPt Data Type Duplicate/2, Difference Inputs1/2  "Y(k-1)"
  Saturation Dynamic/1 -> FixPt Data Type Duplicate/7, Difference Inputs2/1
  up/1 -> delta rise limit/1
  Difference Inputs2/1 -> FixPt Data Type Duplicate/1, Delay Input2/1, Y/1
  delta rise limit/1 -> Saturation Dynamic/1, FixPt Data Type Duplicate/6

== system Aenea_model/AUTOPILOT_MODEL/Misure Sensori/BMP_280/Execution_loop ==
  Input : Inport
  Data Type Conversion : DataTypeConversion  OutDataTypeStr=double
  Data Type Conversion1 : DataTypeConversion  OutDataTypeStr=double
  Data Type Conversion2 : DataTypeConversion  OutDataTypeStr=double
  Data Type Conversion3 : DataTypeConversion  OutDataTypeStr=single
  S-Function Builder : S-Function  FunctionName=BMP280_sfun  SFunctionModules=BMP280_sfun_wrapper  SFunctionDeploymentMode=off  EnableBusSupport=off  mask(S-Function Builder){}
      mask help: Simulink:masks:SFunctionBuilder_MD
      mask init: same as Aenea_model/LOG_DATA_MODEL/S-Function Builder
      settings: CopyFcn=set_param(gcbh,'LinkStatus','none')  OpenFcn=sfunctionwizard(gcbh)
      mask Display: plot(val(:,1),val(:,2)),disp(sys),port_label('input',1,'h_ref'),port_label('output',1,'OAT'),port_label('output',2,'BaroPressure'),port_label('output',3,'BaroAlt')
  T : Outport  VectorParamsAs1DForOutWhenUnconnected=off
  p : Outport  Port=2  VectorParamsAs1DForOutWhenUnconnected=off
  BaroAlt : Outport  Port=3  VectorParamsAs1DForOutWhenUnconnected=off
  wires:
  S-Function Builder/2 -> Data Type Conversion1/1
  S-Function Builder/1 -> Data Type Conversion/1
  S-Function Builder/3 -> Data Type Conversion2/1
  Input/1 -> Data Type Conversion3/1
  Data Type Conversion/1 -> T/1
  Data Type Conversion1/1 -> p/1
  Data Type Conversion2/1 -> BaroAlt/1
  Data Type Conversion3/1 -> S-Function Builder/1

== system Aenea_model/AUTOPILOT_MODEL/Misure Sensori/BMP_280/Subsystem ==
  T : Inport
  Cal_alt : Inport  Port=2
  T_01 : Inport  Port=3
  Constant : Constant  Value=15
  NotEqual : RelationalOperator  Operator=~=  OutDataTypeStr=boolean  RndMeth=Simplest
  Subsystem1 : Subsystem
  Switch : Switch  Criteria=u2 > Threshold
  Switch1 : Switch  Criteria=u2 > Threshold
  T_02 : Outport  VectorParamsAs1DForOutWhenUnconnected=off
  Cal_alt2 : Outport  Port=2  VectorParamsAs1DForOutWhenUnconnected=off
  wires:
  T/1 -> Subsystem1/1(T)
  Cal_alt/1 -> Subsystem1/Enable, Cal_alt2/1
  NotEqual/1 -> Switch1/2
  Subsystem1/1(T_0) -> Switch/2, Switch/1
  Constant/1 -> NotEqual/1
  Switch/1 -> Switch1/3
  Switch1/1 -> T_02/1
  T_01/1 -> Switch/3, Switch1/1, NotEqual/2

== system Aenea_model/AUTOPILOT_MODEL/Misure Sensori/GPS_Venus/Subsystem2 ==
  h : Inport
  fix : Inport  Port=2
  Enable : EnablePort
  Constant : Constant
  Constant1 : Constant  Value=2
  Constant2 : Constant  Value=0
  Constant3 : Constant  Value=3
  Constant4 : Constant  Value=4
  Constant5 : Constant  Value=5
  Constant6 : Constant  Value=6
  Equal{,1..5} (6 alike) : RelationalOperator  Operator===  OutDataTypeStr=boolean  RndMeth=Simplest
  OR : Logic  Operator=OR  Inputs=6  IconShape=distinctive  AllPortsSameDT=off  OutDataTypeStr=boolean
  Switch : Switch  Criteria=u2 > Threshold
  h_to_subtract : Outport  VectorParamsAs1DForOutWhenUnconnected=off
  wires:
  Constant/1 -> Equal/2
  Equal/1 -> OR/1
  h/1 -> Switch/1
  OR/1 -> Switch/2
  Constant2/1 -> Switch/3
  Switch/1 -> h_to_subtract/1
  Constant1/1 -> Equal1/2
  Equal1/1 -> OR/2
  fix/1 -> Equal1/1, Equal2/1, Equal3/1, Equal4/1, Equal5/1, Equal/1
  Constant3/1 -> Equal2/2
  Equal2/1 -> OR/3
  Constant4/1 -> Equal3/2
  Equal3/1 -> OR/4
  Constant5/1 -> Equal4/2
  Equal4/1 -> OR/5
  Constant6/1 -> Equal5/2
  Equal5/1 -> OR/6
